simulink model "untitled"  (R2019a)
settings: Solver=VariableStepAuto  StartTime=0.0  StopTime=1  RelTol=1e-3
values from neighbouring files (symbols this model uses):
  Ts_Control = 5.0000e-05    (= 5e-05)    [Sec_Impedance.m]
  Ts_Power = 5.0000e-05    (= 5e-05)    [Sec_Impedance.m]
undefined symbols (not defined in the file or in its folder): D1, Delta, Ion, Lithium
libraries: powerlib x152, powerlib_meascontrol x65, simulink x14, electricdrivelib x12, simulink_extras x12
(part 3 of 5)

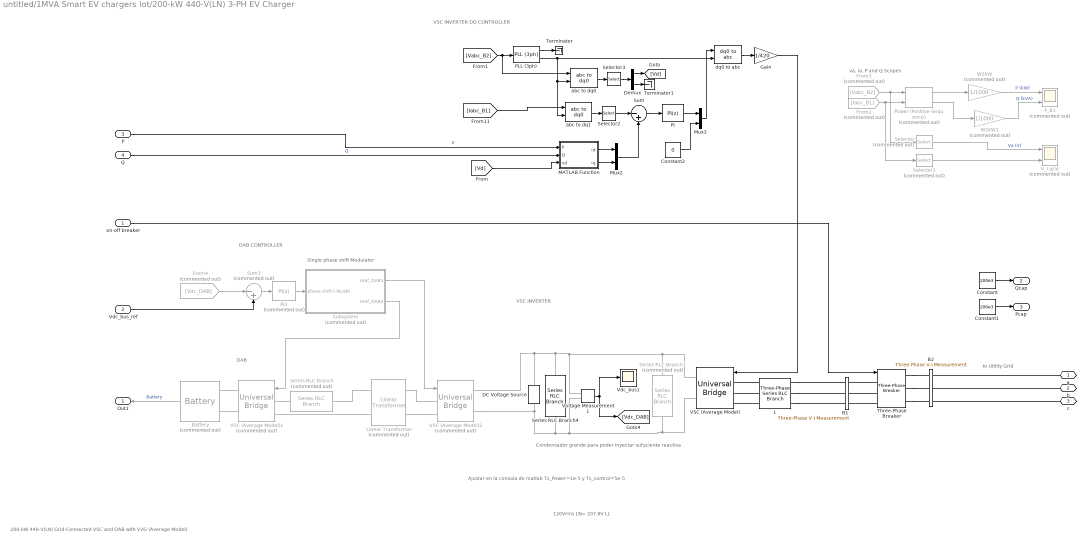
== system untitled/1MVA Smart EV chargers lot/200-kW 440-V(LN) 3-PH EV Charger ==
  note: DAB CONTROLLER
  note: va, ia, P and Q Scopes
  note: 200-kW 440-V(LN) Grid-Connected VSC and DAB with V2G (Average Model)
  note: 120Vrms LN= 207.8V LL
  note: Single phase shift Modulator
  note: Condensador grande para poder inyectar sufuciente reactiva
  note: Ajustar en la consola de matlab Ts_Power=1e-5 y Ts_control=5e-5
  note: to Utility Grid
  note: DAB
  note: VSC INVERTER
  note: VSC INVERTER DQ CONTROLLER
  on-off breaker : Inport
  Vdc_bus_ref : Inport  Port=2
  P : Inport  Port=3
  Q : Inport  Port=4
  B1 : powerlib/Measurements/Three-Phase V-I Measurement  VoltageMeasurement=no  SetLabelV=on  LabelV=Vabc_B1  Vpu=off  VpuLL=off  CurrentMeasurement=yes  SetLabelI=on  LabelI=Iabc_B1  Ipu=off  Pbase=100e6  Vbase=500e3  OutputType=Magnitude  PhasorSimulation=off  PSBequivalent=0
      settings: SourceProductName=Simscape Electrical
  B2 : powerlib/Measurements/Three-Phase V-I Measurement  VoltageMeasurement=phase-to-ground  SetLabelV=on  LabelV=Vabc_B2  Vpu=off  VpuLL=off  CurrentMeasurement=no  SetLabelI=off  LabelI=Iabc_B1  Ipu=off  Pbase=100e6  Vbase=500e3  OutputType=Magnitude  PhasorSimulation=off  PSBequivalent=0
      settings: SourceProductName=Simscape Electrical
  Battery : electricdrivelib/Extra Sources/Battery  Commented=on  BatType=Lithium-Ion  ShowTempParam=off  ThermalPreset=no  ShowAgeParam=off  NomV=380  NomQ=5.4*70  SOC=70  Batt_Tr=20  PresetModel=on  MaxQ=378  MinV=285  FullV=442.3151  Dis_rate=164.3478  R=0.010053  Normal_OP=341.8435  expZone="[410.5466       18.5713]"  current=[6.5 13 32.5]  Units=Time  Tci=20  NomT=20  T2=-30  MaxQ2=4.8  FullV2=7.1  Normal_OP2=5.655  expZone2="[6.58           1]"  Rca=0.6  ti=2000  Dp=0  Neq0=0  Tsim=1e6  Ta1=25  Qeol=5.4*0.9  Reol=0.013333*1.2  Char_age=[2.3478, 3]  Dis_age=[2.3478, 10]  N1=1500  N2=10500  N3=1000  N4=1400  Ta2=45  N5=950
      settings: SourceProductName=Simscape Electrical
  Constant : Constant  Value=200e3
  Constant1 : Constant  Value=200e3
  Constant2 : Constant  Value=0
  DC Voltage Source : powerlib/Electrical Sources/DC Voltage Source  Amplitude=800  Measurements=None
      settings: SourceProductName=Simscape Electrical
  Demux : Demux  Outputs=2
  From2 : From  Commented=on  GotoTag=Iabc_B1  TagVisibility=global
      settings: CloseFcn=tagdialog Close
  From3 : From  Commented=on  GotoTag=Vabc_B2  TagVisibility=global
      settings: CloseFcn=tagdialog Close
  From4 : From  Commented=on  GotoTag=Vdc_DAB
  Gain : Gain  Gain=1/420
  L : powerlib/Elements/Three-Phase Series RLC Branch  LConnTagsString=A|B|C  RConnTagsString=A|B|C  BranchType=RL  Resistance=500e-6*377/50/2  Inductance=1200e-6/2  Capacitance=inf  Measurements=None
      settings: SourceProductName=Simscape Electrical
  Linear Transformer : powerlib/Elements/Linear Transformer  Commented=on  UNITS=SI  NominalPower=[ 250e3 10000 ]  winding1=[400 0.0032 0.4883e-06]  winding2=[800 0.0032 0.4883e-06]  ThreeWindings=off  winding3=[3.15e+05 19845 2105.6]  RmLm=[800 2.1221]  Measurements=None  DataType=on
      settings: SourceProductName=Simscape Electrical
  MATLAB Function : MATLAB Function  TreatAsAtomicUnit=on
  Mux2 : Mux  Inputs=2
  Mux3 : Mux  Inputs=2
  PI : simulink/Continuous/PID Controller  Controller=PI  Form=Parallel  TimeDomain=Discrete-time  SampleTime=Ts_Control  IntegratorMethod=Forward Euler  FilterMethod=Forward Euler  ControllerParametersSource=internal  P=20  I=360  D=0  UseFilter=on  N=100  TunerSelectOption=Transfer Function Based (PID Tuner App)  InitialConditionSource=internal  InitialConditionForIntegrator=0  InitialConditionForFilter=0  DifferentiatorICPrevScaledInput=0  ExternalReset=none  TrackingMode=off  Kt=1  LimitOutput=on  UpperSaturationLimit=800  LowerSaturationLimit=-800  LinearizeAsGain=off  AntiWindupMode=none  Kb=1  POutMin=[]  POutMax=[]  IOutMin=[]  IOutMax=[]  DOutMin=[]  DOutMax=[]  NOutMin=[]  NOutMax=[]  SumOutMin=[]  SumOutMax=[]  SaturationOutMin=[]  SaturationOutMax=[]  PParamMin=[]  PParamMax=[]  IParamMin=[]  IParamMax=[]  DParamMin=[]  DParamMax=[]  NParamMin=[]  NParamMax=[]  KbParamMin=[]  KbParamMax=[]  KtParamMin=[]  KtParamMax=[]  KbOutMin=[]  KbOutMax=[]  KtOutMin=[]  KtOutMax=[]  IntegratorOutMin=[]  IntegratorOutMax=[]  FilterOutMin=[]  FilterOutMax=[]  SumI1OutMin=[]  SumI1OutMax=[]  SumI2OutMin=[]  SumI2OutMax=[]  SumI3OutMin=[]  SumI3OutMax=[]  SumI4OutMin=[]  SumI4OutMax=[]  SumDOutMin=[]  SumDOutMax=[]  DifferentiatorOutMin=[]  DifferentiatorOutMax=[]  FilterDiffOutCoefMin=[]  FilterDiffOutCoefMax=[]  ReciprocalOutMin=[]  ReciprocalOutMax=[]  SumDenOutMin=[]  SumDenOutMax=[]  SumNumOutMin=[]  SumNumOutMax=[]  DivideOutMin=[]  DivideOutMax=[]  IntegratorContinuousStateAttributes=''  IntegratorStateMustResolveToSignalObject=off  IntegratorRTWStateStorageClass=Auto  FilterContinuousStateAttributes=''  FilterStateMustResolveToSignalObject=off  FilterRTWStateStorageClass=Auto  ParallelPVariant=InternalParameters  IdealPVariant=Disabled  IVariant=InternalParameters  DVariant=Disabled  IntegratorVariant=Discrete  SatVariant=Enabled  AWVariant=Passthrough  PCopyVariant=Disabled  TRVariant=Disabled  FdbkBlocksVariant=Forward  IdealPFdbkVariant=Disabled  SatFdbkVariant=Disabled  DerivativeFilterVariant=Disabled  NVariant=Disabled  NCopyVariant=Disabled_SignalSpec  FilterICVariant=Disabled  IntegratorICVariant=InternalICs  ExternalResetVariant=Disabled  TRSumVariant=Passthrough  SumFdbkVariant=Disabled  SumVariant=Sum_PI
  PI3 : simulink/Continuous/PID Controller  Commented=on  Controller=PI  Form=Parallel  TimeDomain=Discrete-time  SampleTime=Ts_Control  IntegratorMethod=Forward Euler  FilterMethod=Forward Euler  ControllerParametersSource=internal  P=4  I=50  D=0  UseFilter=on  N=100  TunerSelectOption=Transfer Function Based (PID Tuner App)  InitialConditionSource=internal  InitialConditionForIntegrator=0  InitialConditionForFilter=0  DifferentiatorICPrevScaledInput=0  ExternalReset=none  TrackingMode=off  Kt=1  LimitOutput=on  UpperSaturationLimit=90  LowerSaturationLimit=-90  LinearizeAsGain=off  AntiWindupMode=none  Kb=1  POutMin=[]  POutMax=[]  IOutMin=[]  IOutMax=[]  DOutMin=[]  DOutMax=[]  NOutMin=[]  NOutMax=[]  SumOutMin=[]  SumOutMax=[]  SaturationOutMin=[]  SaturationOutMax=[]  PParamMin=[]  PParamMax=[]  IParamMin=[]  IParamMax=[]  DParamMin=[]  DParamMax=[]  NParamMin=[]  NParamMax=[]  KbParamMin=[]  KbParamMax=[]  KtParamMin=[]  KtParamMax=[]  KbOutMin=[]  KbOutMax=[]  KtOutMin=[]  KtOutMax=[]  IntegratorOutMin=[]  IntegratorOutMax=[]  FilterOutMin=[]  FilterOutMax=[]  SumI1OutMin=[]  SumI1OutMax=[]  SumI2OutMin=[]  SumI2OutMax=[]  SumI3OutMin=[]  SumI3OutMax=[]  SumI4OutMin=[]  SumI4OutMax=[]  SumDOutMin=[]  SumDOutMax=[]  DifferentiatorOutMin=[]  DifferentiatorOutMax=[]  FilterDiffOutCoefMin=[]  FilterDiffOutCoefMax=[]  ReciprocalOutMin=[]  ReciprocalOutMax=[]  SumDenOutMin=[]  SumDenOutMax=[]  SumNumOutMin=[]  SumNumOutMax=[]  DivideOutMin=[]  DivideOutMax=[]  IntegratorContinuousStateAttributes=''  IntegratorStateMustResolveToSignalObject=off  IntegratorRTWStateStorageClass=Auto  FilterContinuousStateAttributes=''  FilterStateMustResolveToSignalObject=off  FilterRTWStateStorageClass=Auto  ParallelPVariant=InternalParameters  IdealPVariant=Disabled  IVariant=InternalParameters  DVariant=Disabled  IntegratorVariant=Discrete  SatVariant=Enabled  AWVariant=Passthrough  PCopyVariant=Disabled  TRVariant=Disabled  FdbkBlocksVariant=Forward  IdealPFdbkVariant=Disabled  SatFdbkVariant=Disabled  DerivativeFilterVariant=Disabled  NVariant=Disabled  NCopyVariant=Disabled_SignalSpec  FilterICVariant=Disabled  IntegratorICVariant=InternalICs  ExternalResetVariant=Disabled  TRSumVariant=Passthrough  SumFdbkVariant=Disabled  SumVariant=Sum_PI
  PLL (3ph) : powerlib_meascontrol/PLL/PLL (3ph)  Fmin=58  Par_Init="[-0.57  60]"  ParK=[180, 3200, 1]  TcD=1e-4  MaxRateChangeFreq=12  FilterCutOffFreq=25  Ts=Ts_Power  AGC=on
      settings: SourceProductName=Simscape Electrical
  P_B1 : Scope  Commented=on  NumInputPorts=2
  Power (Positive-Sequence) : powerlib_meascontrol/Measurements/Power (Positive-Sequence)  Commented=on  Freq=60  Vinit=[0, 0]  Iinit=[0, 0]  Ts=Ts_Control
      settings: SourceProductName=Simscape Electrical  SourceProductBaseCode=PS
  Selector : Selector  Commented=on  InputPortWidth=3  IndexOptions=Index vector (dialog)  Indices=[1]  OutputSizes=1
  Selector1 : Selector  Commented=on  InputPortWidth=3  IndexOptions=Index vector (dialog)  Indices=[1]  OutputSizes=1
  Selector2 : Selector  InputPortWidth=3  IndexOptions=Index vector (dialog)  Indices=[1 2]  OutputSizes=1
  Selector3 : Selector  InputPortWidth=3  IndexOptions=Index vector (dialog)  Indices=[1 2]  OutputSizes=1
  Series RLC Branch : powerlib/Elements/Series RLC Branch  Commented=on  LConnTagsString=__new0  RConnTagsString=__new0  BranchType=L  Resistance=1  Inductance=1.5e-6  SetiL0=off  InitialCurrent=0  Capacitance=1e-6  Setx0=off  InitialVoltage=0  Measurements=None
      settings: SourceProductName=Simscape Electrical
  Series RLC Branch1 : powerlib/Elements/Series RLC Branch  Commented=on  LConnTagsString=__new0  RConnTagsString=__new0  BranchType=R  Resistance=3.2  Inductance=1e-3  SetiL0=off  InitialCurrent=0  Capacitance=1200e-6  Setx0=off  InitialVoltage=400  Measurements=None
      settings: SourceProductName=Simscape Electrical
  Series RLC Branch4 : powerlib/Elements/Series RLC Branch  LConnTagsString=__new0  RConnTagsString=__new0  BranchType=RC  Resistance=1e-7  Inductance=1e-3  SetiL0=off  InitialCurrent=0  Capacitance=3600e-6  Setx0=off  InitialVoltage=400  Measurements=None
      settings: SourceProductName=Simscape Electrical
  Subsystem : Subsystem  Commented=on
  Sum : Sum  Inputs=|-+
  Sum3 : Sum  Commented=on  Inputs=|-+
  Terminator : Terminator
  Terminator1 : Terminator
  Three-Phase Breaker : powerlib/Elements/Three-Phase Breaker  InitialState=open  SwitchA=on  SwitchB=on  SwitchC=on  SwitchTimes="[1/6  5/6]"  External=on  BreakerResistance=0.01e-3  SnubberResistance=30  SnubberCapacitance=20e-6  Measurements=None
      settings: SourceProductName=Simscape Electrical
  VSC (Average Model) : powerlib/Power Electronics/Universal Bridge  Arms=3  SnubberResistance=1e5  SnubberCapacitance=inf  Device=Average-model based VSC  Ron=1e-3  Lon=0  ForwardVoltages="[  0  0  ]"  ForwardVoltage=0  GTOparameters=[ 10e-6 , 20e-6 ]  IGBTparameters=[ 1e-6 , 2e-6 ]  Measurements=None  Measurements_2=None  converterType=Rectifier
      settings: SourceProductName=Simscape Electrical
  VSC (Average Model)1 : powerlib/Power Electronics/Universal Bridge  Commented=on  Arms=2  SnubberResistance=1e5  SnubberCapacitance=inf  Device=Average-model based VSC  Ron=1e-3  Lon=0  ForwardVoltages="[  0  0  ]"  ForwardVoltage=0  GTOparameters=[ 10e-6 , 20e-6 ]  IGBTparameters=[ 1e-6 , 2e-6 ]  Measurements=None  Measurements_2=None  converterType=Rectifier
      settings: SourceProductName=Simscape Electrical
  VSC (Average Model)2 : powerlib/Power Electronics/Universal Bridge  Commented=on  Arms=2  SnubberResistance=1e5  SnubberCapacitance=inf  Device=Average-model based VSC  Ron=1e-3  Lon=0  ForwardVoltages="[  0  0  ]"  ForwardVoltage=0  GTOparameters=[ 10e-6 , 20e-6 ]  IGBTparameters=[ 1e-6 , 2e-6 ]  Measurements=None  Measurements_2=None  converterType=Rectifier
      settings: SourceProductName=Simscape Electrical
  V_I grid : Scope  Commented=on  NumInputPorts=2
  Vdc_bus1 : Scope
  Voltage Measurement1 : powerlib/Measurements/Voltage Measurement  PhasorSimulation=off  OutputType=Complex  PSBequivalent=0
      settings: SourceProductName=Simscape Electrical
  W2kW : Gain  Commented=on  Gain=1/1000
  W2kW1 : Gain  Commented=on  Gain=1/1000
  abc to dq0 : powerlib_meascontrol/Transformations/abc to dq0  Alignment=90 degrees behind phase A axis
      settings: SourceProductName=Simscape Electrical
  abc to dq1 : powerlib_meascontrol/Transformations/abc to dq0  Alignment=90 degrees behind phase A axis
      settings: SourceProductName=Simscape Electrical
  dq0 to abc : powerlib_meascontrol/Transformations/dq0 to abc  Alignment=90 degrees behind phase A axis
      settings: SourceProductName=Simscape Electrical
  a : PMIOPort  Side=Right
  b : PMIOPort  Port=2  Side=Right
  c : PMIOPort  Port=3  Side=Right
  Out1 : Outport
  Qcap : Outport  Port=2
  Pcap : Outport  Port=3
  wires:
  PLL (3ph)/2 -> abc to dq1/2, abc to dq0/2, dq0 to abc/2
  Subsystem/1(Uref_DAB1) -> VSC (Average Model)2/1
  PI/1 -> Mux3/1
  Selector/1 -> V_I grid/1  "Va (V)"
  dq0 to abc/1 -> Gain/1
  Vdc_bus_ref/1 -> Sum3/2
  PLL (3ph)/1 -> Terminator/1
  From2/1 -> Selector1/1, Power (Positive-Sequence)/2
  abc to dq1/1 -> Selector2/1
  Mux3/1 -> dq0 to abc/1
  Gain/1 -> VSC (Average Model)/1
  W2kW1/1 -> P_B1/2  "Q (kVA)"
  Selector2/1 -> Sum/1
  Sum/1 -> PI/1
  [Vabc_B2] -> abc to dq0/1, PLL (3ph)/1
  Subsystem/2(Uref_DAB2) -> VSC (Average Model)1/1
  Sum3/1 -> PI3/1
  W2kW/1 -> P_B1/1  "P (kW)"
  Constant2/1 -> Mux3/2
  PI3/1 -> Subsystem/1(phase shift (-90,90))
  Selector3/1 -> Demux/1
  From3/1 -> Selector/1, Power (Positive-Sequence)/1
  Selector1/1 -> V_I grid/2
  From4/1 -> Sum3/1
  abc to dq0/1 -> Selector3/1
  Power (Positive-Sequence)/1 -> W2kW/1
  Voltage Measurement1/1 -> Vdc_bus1/1, [Vdc_DAB]
  Mux2/1 -> Sum/2
  [Iabc_B1] -> abc to dq1/1
  Power (Positive-Sequence)/2 -> W2kW1/1
  Battery/1 -> Out1/1  "Battery"
  on-off breaker/1 -> Three-Phase Breaker/1
  Demux/2 -> Terminator1/1
  Demux/1 -> [Vd]
  MATLAB Function/1(id) -> Mux2/1
  MATLAB Function/2(iq) -> Mux2/2
  [Vd] -> MATLAB Function/3(vd)
  P/1 -> MATLAB Function/1(P)  "P"
  Q/1 -> MATLAB Function/2(Q)  "Q"
  Constant1/1 -> Pcap/1
  Constant/1 -> Qcap/1
  connections:
  Battery/LConn1 -- VSC (Average Model)1/RConn1
  Three-Phase Breaker/LConn1 -- B1/RConn1
  Three-Phase Breaker/RConn2 -- B2/LConn2
  VSC (Average Model)2/RConn2 -- DC Voltage Source/LConn1 -- Series RLC Branch4/RConn1 -- Voltage Measurement1/LConn2 -- VSC (Average Model)/RConn2 -- Series RLC Branch1/RConn1
  L/RConn3 -- B1/LConn3
  L/LConn1 -- VSC (Average Model)/LConn1
  L/RConn1 -- B1/LConn1
  L/LConn2 -- VSC (Average Model)/LConn2
  VSC (Average Model)2/RConn1 -- Series RLC Branch1/LConn1 -- VSC (Average Model)/RConn1 -- Voltage Measurement1/LConn1 -- Series RLC Branch4/LConn1 -- DC Voltage Source/RConn1
  Series RLC Branch/RConn1 -- Linear Transformer/LConn1
  Linear Transformer/LConn2 -- VSC (Average Model)1/LConn2
  Three-Phase Breaker/LConn2 -- B1/RConn2
  VSC (Average Model)1/RConn2 -- Battery/LConn2
  Three-Phase Breaker/RConn3 -- B2/LConn3
  Three-Phase Breaker/RConn1 -- B2/LConn1
  Linear Transformer/RConn1 -- VSC (Average Model)2/LConn1
  Linear Transformer/RConn2 -- VSC (Average Model)2/LConn2
  c/RConn1 -- B2/RConn3
  Series RLC Branch/LConn1 -- VSC (Average Model)1/LConn1
  L/RConn2 -- B1/LConn2
  L/LConn3 -- VSC (Average Model)/LConn3
  Three-Phase Breaker/LConn3 -- B1/RConn3
  b/RConn1 -- B2/RConn2
  a/RConn1 -- B2/RConn1

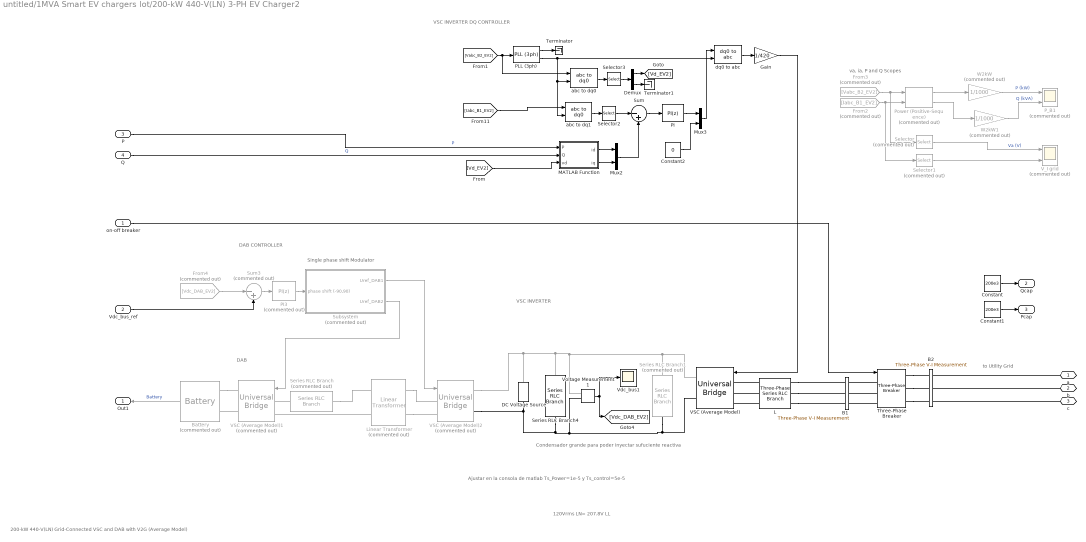
== system untitled/1MVA Smart EV chargers lot/200-kW 440-V(LN) 3-PH EV Charger2 ==
  note: DAB CONTROLLER
  note: va, ia, P and Q Scopes
  note: 200-kW 440-V(LN) Grid-Connected VSC and DAB with V2G (Average Model)
  note: 120Vrms LN= 207.8V LL
  note: Single phase shift Modulator
  note: Condensador grande para poder inyectar sufuciente reactiva
  note: Ajustar en la consola de matlab Ts_Power=1e-5 y Ts_control=5e-5
  note: to Utility Grid
  note: DAB
  note: VSC INVERTER
  note: VSC INVERTER DQ CONTROLLER
  on-off breaker : Inport
  Vdc_bus_ref : Inport  Port=2
  P : Inport  Port=3
  Q : Inport  Port=4
  B1 : powerlib/Measurements/Three-Phase V-I Measurement  VoltageMeasurement=no  SetLabelV=on  LabelV=Vabc_B1  Vpu=off  VpuLL=off  CurrentMeasurement=yes  SetLabelI=on  LabelI=Iabc_B1_EV2  Ipu=off  Pbase=100e6  Vbase=500e3  OutputType=Magnitude  PhasorSimulation=off  PSBequivalent=0
      settings: SourceProductName=Simscape Electrical
  B2 : powerlib/Measurements/Three-Phase V-I Measurement  VoltageMeasurement=phase-to-ground  SetLabelV=on  LabelV=Vabc_B2_EV2  Vpu=off  VpuLL=off  CurrentMeasurement=no  SetLabelI=off  LabelI=Iabc_B1  Ipu=off  Pbase=100e6  Vbase=500e3  OutputType=Magnitude  PhasorSimulation=off  PSBequivalent=0
      settings: SourceProductName=Simscape Electrical
  Battery : electricdrivelib/Extra Sources/Battery  Commented=on  BatType=Lithium-Ion  ShowTempParam=off  ThermalPreset=no  ShowAgeParam=off  NomV=380  NomQ=5.4*70  SOC=70  Batt_Tr=20  PresetModel=on  MaxQ=378  MinV=285  FullV=442.3151  Dis_rate=164.3478  R=0.010053  Normal_OP=341.8435  expZone="[410.5466       18.5713]"  current=[6.5 13 32.5]  Units=Time  Tci=20  NomT=20  T2=-30  MaxQ2=4.8  FullV2=7.1  Normal_OP2=5.655  expZone2="[6.58           1]"  Rca=0.6  ti=2000  Dp=0  Neq0=0  Tsim=1e6  Ta1=25  Qeol=5.4*0.9  Reol=0.013333*1.2  Char_age=[2.3478, 3]  Dis_age=[2.3478, 10]  N1=1500  N2=10500  N3=1000  N4=1400  Ta2=45  N5=950
      settings: SourceProductName=Simscape Electrical
  Constant : Constant  Value=200e3
  Constant1 : Constant  Value=200e3
  Constant2 : Constant  Value=0
  DC Voltage Source : powerlib/Electrical Sources/DC Voltage Source  Amplitude=800  Measurements=None
      settings: SourceProductName=Simscape Electrical
  Demux : Demux  Outputs=2
  From2 : From  Commented=on  GotoTag=Iabc_B1_EV2  TagVisibility=global
      settings: CloseFcn=tagdialog Close
  From3 : From  Commented=on  GotoTag=Vabc_B2_EV2  TagVisibility=global
      settings: CloseFcn=tagdialog Close
  From4 : From  Commented=on  GotoTag=Vdc_DAB_EV2
  Gain : Gain  Gain=1/420
  L : powerlib/Elements/Three-Phase Series RLC Branch  LConnTagsString=A|B|C  RConnTagsString=A|B|C  BranchType=RL  Resistance=500e-6*377/50/2  Inductance=1200e-6/2  Capacitance=inf  Measurements=None
      settings: SourceProductName=Simscape Electrical
  Linear Transformer : powerlib/Elements/Linear Transformer  Commented=on  UNITS=SI  NominalPower=[ 250e3 10000 ]  winding1=[400 0.0032 0.4883e-06]  winding2=[800 0.0032 0.4883e-06]  ThreeWindings=off  winding3=[3.15e+05 19845 2105.6]  RmLm=[800 2.1221]  Measurements=None  DataType=on
      settings: SourceProductName=Simscape Electrical
  MATLAB Function : MATLAB Function  TreatAsAtomicUnit=on
  Mux2 : Mux  Inputs=2
  Mux3 : Mux  Inputs=2
  PI : simulink/Continuous/PID Controller  Controller=PI  Form=Parallel  TimeDomain=Discrete-time  SampleTime=Ts_Control  IntegratorMethod=Forward Euler  FilterMethod=Forward Euler  ControllerParametersSource=internal  P=20  I=360  D=0  UseFilter=on  N=100  TunerSelectOption=Transfer Function Based (PID Tuner App)  InitialConditionSource=internal  InitialConditionForIntegrator=0  InitialConditionForFilter=0  DifferentiatorICPrevScaledInput=0  ExternalReset=none  TrackingMode=off  Kt=1  LimitOutput=on  UpperSaturationLimit=800  LowerSaturationLimit=-800  LinearizeAsGain=off  AntiWindupMode=none  Kb=1  POutMin=[]  POutMax=[]  IOutMin=[]  IOutMax=[]  DOutMin=[]  DOutMax=[]  NOutMin=[]  NOutMax=[]  SumOutMin=[]  SumOutMax=[]  SaturationOutMin=[]  SaturationOutMax=[]  PParamMin=[]  PParamMax=[]  IParamMin=[]  IParamMax=[]  DParamMin=[]  DParamMax=[]  NParamMin=[]  NParamMax=[]  KbParamMin=[]  KbParamMax=[]  KtParamMin=[]  KtParamMax=[]  KbOutMin=[]  KbOutMax=[]  KtOutMin=[]  KtOutMax=[]  IntegratorOutMin=[]  IntegratorOutMax=[]  FilterOutMin=[]  FilterOutMax=[]  SumI1OutMin=[]  SumI1OutMax=[]  SumI2OutMin=[]  SumI2OutMax=[]  SumI3OutMin=[]  SumI3OutMax=[]  SumI4OutMin=[]  SumI4OutMax=[]  SumDOutMin=[]  SumDOutMax=[]  DifferentiatorOutMin=[]  DifferentiatorOutMax=[]  FilterDiffOutCoefMin=[]  FilterDiffOutCoefMax=[]  ReciprocalOutMin=[]  ReciprocalOutMax=[]  SumDenOutMin=[]  SumDenOutMax=[]  SumNumOutMin=[]  SumNumOutMax=[]  DivideOutMin=[]  DivideOutMax=[]  IntegratorContinuousStateAttributes=''  IntegratorStateMustResolveToSignalObject=off  IntegratorRTWStateStorageClass=Auto  FilterContinuousStateAttributes=''  FilterStateMustResolveToSignalObject=off  FilterRTWStateStorageClass=Auto  ParallelPVariant=InternalParameters  IdealPVariant=Disabled  IVariant=InternalParameters  DVariant=Disabled  IntegratorVariant=Discrete  SatVariant=Enabled  AWVariant=Passthrough  PCopyVariant=Disabled  TRVariant=Disabled  FdbkBlocksVariant=Forward  IdealPFdbkVariant=Disabled  SatFdbkVariant=Disabled  DerivativeFilterVariant=Disabled  NVariant=Disabled  NCopyVariant=Disabled_SignalSpec  FilterICVariant=Disabled  IntegratorICVariant=InternalICs  ExternalResetVariant=Disabled  TRSumVariant=Passthrough  SumFdbkVariant=Disabled  SumVariant=Sum_PI
  PI3 : simulink/Continuous/PID Controller  Commented=on  Controller=PI  Form=Parallel  TimeDomain=Discrete-time  SampleTime=Ts_Control  IntegratorMethod=Forward Euler  FilterMethod=Forward Euler  ControllerParametersSource=internal  P=4  I=50  D=0  UseFilter=on  N=100  TunerSelectOption=Transfer Function Based (PID Tuner App)  InitialConditionSource=internal  InitialConditionForIntegrator=0  InitialConditionForFilter=0  DifferentiatorICPrevScaledInput=0  ExternalReset=none  TrackingMode=off  Kt=1  LimitOutput=on  UpperSaturationLimit=90  LowerSaturationLimit=-90  LinearizeAsGain=off  AntiWindupMode=none  Kb=1  POutMin=[]  POutMax=[]  IOutMin=[]  IOutMax=[]  DOutMin=[]  DOutMax=[]  NOutMin=[]  NOutMax=[]  SumOutMin=[]  SumOutMax=[]  SaturationOutMin=[]  SaturationOutMax=[]  PParamMin=[]  PParamMax=[]  IParamMin=[]  IParamMax=[]  DParamMin=[]  DParamMax=[]  NParamMin=[]  NParamMax=[]  KbParamMin=[]  KbParamMax=[]  KtParamMin=[]  KtParamMax=[]  KbOutMin=[]  KbOutMax=[]  KtOutMin=[]  KtOutMax=[]  IntegratorOutMin=[]  IntegratorOutMax=[]  FilterOutMin=[]  FilterOutMax=[]  SumI1OutMin=[]  SumI1OutMax=[]  SumI2OutMin=[]  SumI2OutMax=[]  SumI3OutMin=[]  SumI3OutMax=[]  SumI4OutMin=[]  SumI4OutMax=[]  SumDOutMin=[]  SumDOutMax=[]  DifferentiatorOutMin=[]  DifferentiatorOutMax=[]  FilterDiffOutCoefMin=[]  FilterDiffOutCoefMax=[]  ReciprocalOutMin=[]  ReciprocalOutMax=[]  SumDenOutMin=[]  SumDenOutMax=[]  SumNumOutMin=[]  SumNumOutMax=[]  DivideOutMin=[]  DivideOutMax=[]  IntegratorContinuousStateAttributes=''  IntegratorStateMustResolveToSignalObject=off  IntegratorRTWStateStorageClass=Auto  FilterContinuousStateAttributes=''  FilterStateMustResolveToSignalObject=off  FilterRTWStateStorageClass=Auto  ParallelPVariant=InternalParameters  IdealPVariant=Disabled  IVariant=InternalParameters  DVariant=Disabled  IntegratorVariant=Discrete  SatVariant=Enabled  AWVariant=Passthrough  PCopyVariant=Disabled  TRVariant=Disabled  FdbkBlocksVariant=Forward  IdealPFdbkVariant=Disabled  SatFdbkVariant=Disabled  DerivativeFilterVariant=Disabled  NVariant=Disabled  NCopyVariant=Disabled_SignalSpec  FilterICVariant=Disabled  IntegratorICVariant=InternalICs  ExternalResetVariant=Disabled  TRSumVariant=Passthrough  SumFdbkVariant=Disabled  SumVariant=Sum_PI
  PLL (3ph) : powerlib_meascontrol/PLL/PLL (3ph)  Fmin=55  Par_Init="[-0.57  60]"  ParK=[180, 3200, 1]  TcD=1e-4  MaxRateChangeFreq=12  FilterCutOffFreq=25  Ts=Ts_Power  AGC=on
      settings: SourceProductName=Simscape Electrical
  P_B1 : Scope  Commented=on  NumInputPorts=2
  Power (Positive-Sequence) : powerlib_meascontrol/Measurements/Power (Positive-Sequence)  Commented=on  Freq=60  Vinit=[0, 0]  Iinit=[0, 0]  Ts=Ts_Control
      settings: SourceProductName=Simscape Electrical  SourceProductBaseCode=PS
  Selector : Selector  Commented=on  InputPortWidth=3  IndexOptions=Index vector (dialog)  Indices=[1]  OutputSizes=1
  Selector1 : Selector  Commented=on  InputPortWidth=3  IndexOptions=Index vector (dialog)  Indices=[1]  OutputSizes=1
  Selector2 : Selector  InputPortWidth=3  IndexOptions=Index vector (dialog)  Indices=[1 2]  OutputSizes=1
  Selector3 : Selector  InputPortWidth=3  IndexOptions=Index vector (dialog)  Indices=[1 2]  OutputSizes=1
  Series RLC Branch : powerlib/Elements/Series RLC Branch  Commented=on  LConnTagsString=__new0  RConnTagsString=__new0  BranchType=L  Resistance=1  Inductance=1.5e-6  SetiL0=off  InitialCurrent=0  Capacitance=1e-6  Setx0=off  InitialVoltage=0  Measurements=None
      settings: SourceProductName=Simscape Electrical
  Series RLC Branch1 : powerlib/Elements/Series RLC Branch  Commented=on  LConnTagsString=__new0  RConnTagsString=__new0  BranchType=R  Resistance=3.2  Inductance=1e-3  SetiL0=off  InitialCurrent=0  Capacitance=1200e-6  Setx0=off  InitialVoltage=400  Measurements=None
      settings: SourceProductName=Simscape Electrical
  Series RLC Branch4 : powerlib/Elements/Series RLC Branch  LConnTagsString=__new0  RConnTagsString=__new0  BranchType=RC  Resistance=1e-7  Inductance=1e-3  SetiL0=off  InitialCurrent=0  Capacitance=3600e-6  Setx0=off  InitialVoltage=400  Measurements=None
      settings: SourceProductName=Simscape Electrical
  Subsystem : Subsystem  Commented=on
  Sum : Sum  Inputs=|-+
  Sum3 : Sum  Commented=on  Inputs=|-+
  Terminator : Terminator
  Terminator1 : Terminator
  Three-Phase Breaker : powerlib/Elements/Three-Phase Breaker  InitialState=open  SwitchA=on  SwitchB=on  SwitchC=on  SwitchTimes="[1/6  5/6]"  External=on  BreakerResistance=0.01e-3  SnubberResistance=30  SnubberCapacitance=20e-6  Measurements=None
      settings: SourceProductName=Simscape Electrical
  VSC (Average Model) : powerlib/Power Electronics/Universal Bridge  Arms=3  SnubberResistance=1e5  SnubberCapacitance=inf  Device=Average-model based VSC  Ron=1e-3  Lon=0  ForwardVoltages="[  0  0  ]"  ForwardVoltage=0  GTOparameters=[ 10e-6 , 20e-6 ]  IGBTparameters=[ 1e-6 , 2e-6 ]  Measurements=None  Measurements_2=None  converterType=Rectifier
      settings: SourceProductName=Simscape Electrical
  VSC (Average Model)1 : powerlib/Power Electronics/Universal Bridge  Commented=on  Arms=2  SnubberResistance=1e5  SnubberCapacitance=inf  Device=Average-model based VSC  Ron=1e-3  Lon=0  ForwardVoltages="[  0  0  ]"  ForwardVoltage=0  GTOparameters=[ 10e-6 , 20e-6 ]  IGBTparameters=[ 1e-6 , 2e-6 ]  Measurements=None  Measurements_2=None  converterType=Rectifier
      settings: SourceProductName=Simscape Electrical
  VSC (Average Model)2 : powerlib/Power Electronics/Universal Bridge  Commented=on  Arms=2  SnubberResistance=1e5  SnubberCapacitance=inf  Device=Average-model based VSC  Ron=1e-3  Lon=0  ForwardVoltages="[  0  0  ]"  ForwardVoltage=0  GTOparameters=[ 10e-6 , 20e-6 ]  IGBTparameters=[ 1e-6 , 2e-6 ]  Measurements=None  Measurements_2=None  converterType=Rectifier
      settings: SourceProductName=Simscape Electrical
  V_I grid : Scope  Commented=on  NumInputPorts=2
  Vdc_bus1 : Scope
  Voltage Measurement1 : powerlib/Measurements/Voltage Measurement  PhasorSimulation=off  OutputType=Complex  PSBequivalent=0
      settings: SourceProductName=Simscape Electrical
  W2kW : Gain  Commented=on  Gain=1/1000
  W2kW1 : Gain  Commented=on  Gain=1/1000
  abc to dq0 : powerlib_meascontrol/Transformations/abc to dq0  Alignment=90 degrees behind phase A axis
      settings: SourceProductName=Simscape Electrical
  abc to dq1 : powerlib_meascontrol/Transformations/abc to dq0  Alignment=90 degrees behind phase A axis
      settings: SourceProductName=Simscape Electrical
  dq0 to abc : powerlib_meascontrol/Transformations/dq0 to abc  Alignment=90 degrees behind phase A axis
      settings: SourceProductName=Simscape Electrical
  a : PMIOPort  Side=Right
  b : PMIOPort  Port=2  Side=Right
  c : PMIOPort  Port=3  Side=Right
  Out1 : Outport
  Qcap : Outport  Port=2
  Pcap : Outport  Port=3
  wires:
  PLL (3ph)/2 -> abc to dq1/2, abc to dq0/2, dq0 to abc/2
  Subsystem/1(Uref_DAB1) -> VSC (Average Model)2/1
  PI/1 -> Mux3/1
  Selector/1 -> V_I grid/1  "Va (V)"
  dq0 to abc/1 -> Gain/1
  Vdc_bus_ref/1 -> Sum3/2
  PLL (3ph)/1 -> Terminator/1
  From2/1 -> Selector1/1, Power (Positive-Sequence)/2
  abc to dq1/1 -> Selector2/1
  Mux3/1 -> dq0 to abc/1
  Gain/1 -> VSC (Average Model)/1
  W2kW1/1 -> P_B1/2  "Q (kVA)"
  Selector2/1 -> Sum/1
  Sum/1 -> PI/1
  [Vabc_B2_EV2] -> abc to dq0/1, PLL (3ph)/1
  Subsystem/2(Uref_DAB2) -> VSC (Average Model)1/1
  Sum3/1 -> PI3/1
  W2kW/1 -> P_B1/1  "P (kW)"
  Constant2/1 -> Mux3/2
  PI3/1 -> Subsystem/1(phase shift (-90,90))
  Selector3/1 -> Demux/1
  From3/1 -> Selector/1, Power (Positive-Sequence)/1
  Selector1/1 -> V_I grid/2
  From4/1 -> Sum3/1
  abc to dq0/1 -> Selector3/1
  Power (Positive-Sequence)/1 -> W2kW/1
  Voltage Measurement1/1 -> Vdc_bus1/1, [Vdc_DAB_EV2]
  Mux2/1 -> Sum/2
  [Iabc_B1_EV2] -> abc to dq1/1
  Power (Positive-Sequence)/2 -> W2kW1/1
  Battery/1 -> Out1/1  "Battery"
  on-off breaker/1 -> Three-Phase Breaker/1
  Demux/2 -> Terminator1/1
  Demux/1 -> [Vd_EV2]
  MATLAB Function/1(id) -> Mux2/1
  MATLAB Function/2(iq) -> Mux2/2
  [Vd_EV2] -> MATLAB Function/3(vd)
  P/1 -> MATLAB Function/1(P)  "P"
  Q/1 -> MATLAB Function/2(Q)  "Q"
  Constant1/1 -> Pcap/1
  Constant/1 -> Qcap/1
  connections:
  Battery/LConn1 -- VSC (Average Model)1/RConn1
  Three-Phase Breaker/LConn1 -- B1/RConn1
  Three-Phase Breaker/RConn2 -- B2/LConn2
  VSC (Average Model)/RConn2 -- Series RLC Branch1/RConn1 -- VSC (Average Model)2/RConn2 -- DC Voltage Source/LConn1 -- Series RLC Branch4/RConn1 -- Voltage Measurement1/LConn2
  L/RConn3 -- B1/LConn3
  L/LConn1 -- VSC (Average Model)/LConn1
  L/RConn1 -- B1/LConn1
  L/LConn2 -- VSC (Average Model)/LConn2
  Series RLC Branch1/LConn1 -- VSC (Average Model)/RConn1 -- DC Voltage Source/RConn1 -- VSC (Average Model)2/RConn1 -- Series RLC Branch4/LConn1 -- Voltage Measurement1/LConn1
  Series RLC Branch/RConn1 -- Linear Transformer/LConn1
  Linear Transformer/LConn2 -- VSC (Average Model)1/LConn2
  Three-Phase Breaker/LConn2 -- B1/RConn2
  VSC (Average Model)1/RConn2 -- Battery/LConn2
  Three-Phase Breaker/RConn3 -- B2/LConn3
  Three-Phase Breaker/RConn1 -- B2/LConn1
  Linear Transformer/RConn1 -- VSC (Average Model)2/LConn1
  Linear Transformer/RConn2 -- VSC (Average Model)2/LConn2
  c/RConn1 -- B2/RConn3
  Series RLC Branch/LConn1 -- VSC (Average Model)1/LConn1
  L/RConn2 -- B1/LConn2
  L/LConn3 -- VSC (Average Model)/LConn3
  Three-Phase Breaker/LConn3 -- B1/RConn3
  b/RConn1 -- B2/RConn2
  a/RConn1 -- B2/RConn1

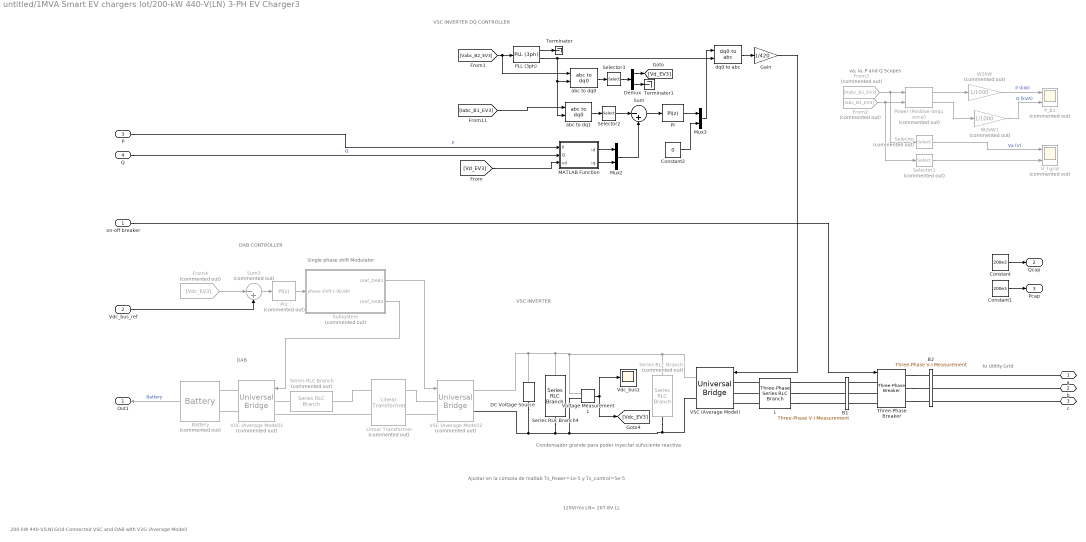
== system untitled/1MVA Smart EV chargers lot/200-kW 440-V(LN) 3-PH EV Charger3 ==
  note: DAB CONTROLLER
  note: va, ia, P and Q Scopes
  note: 200-kW 440-V(LN) Grid-Connected VSC and DAB with V2G (Average Model)
  note: 120Vrms LN= 207.8V LL
  note: Single phase shift Modulator
  note: Condensador grande para poder inyectar sufuciente reactiva
  note: Ajustar en la consola de matlab Ts_Power=1e-5 y Ts_control=5e-5
  note: to Utility Grid
  note: DAB
  note: VSC INVERTER
  note: VSC INVERTER DQ CONTROLLER
  on-off breaker : Inport
  Vdc_bus_ref : Inport  Port=2
  P : Inport  Port=3
  Q : Inport  Port=4
  B1 : powerlib/Measurements/Three-Phase V-I Measurement  VoltageMeasurement=no  SetLabelV=on  LabelV=Vabc_B1  Vpu=off  VpuLL=off  CurrentMeasurement=yes  SetLabelI=on  LabelI=Iabc_B1_EV3  Ipu=off  Pbase=100e6  Vbase=500e3  OutputType=Magnitude  PhasorSimulation=off  PSBequivalent=0
      settings: SourceProductName=Simscape Electrical
  B2 : powerlib/Measurements/Three-Phase V-I Measurement  VoltageMeasurement=phase-to-ground  SetLabelV=on  LabelV=Vabc_B2_EV3  Vpu=off  VpuLL=off  CurrentMeasurement=no  SetLabelI=off  LabelI=Iabc_B1  Ipu=off  Pbase=100e6  Vbase=500e3  OutputType=Magnitude  PhasorSimulation=off  PSBequivalent=0
      settings: SourceProductName=Simscape Electrical
  Battery : electricdrivelib/Extra Sources/Battery  Commented=on  BatType=Lithium-Ion  ShowTempParam=off  ThermalPreset=no  ShowAgeParam=off  NomV=380  NomQ=5.4*70  SOC=70  Batt_Tr=20  PresetModel=on  MaxQ=378  MinV=285  FullV=442.3151  Dis_rate=164.3478  R=0.010053  Normal_OP=341.8435  expZone="[410.5466       18.5713]"  current=[6.5 13 32.5]  Units=Time  Tci=20  NomT=20  T2=-30  MaxQ2=4.8  FullV2=7.1  Normal_OP2=5.655  expZone2="[6.58           1]"  Rca=0.6  ti=2000  Dp=0  Neq0=0  Tsim=1e6  Ta1=25  Qeol=5.4*0.9  Reol=0.013333*1.2  Char_age=[2.3478, 3]  Dis_age=[2.3478, 10]  N1=1500  N2=10500  N3=1000  N4=1400  Ta2=45  N5=950
      settings: SourceProductName=Simscape Electrical
  Constant : Constant  Value=200e3
  Constant1 : Constant  Value=200e3
  Constant2 : Constant  Value=0
  DC Voltage Source : powerlib/Electrical Sources/DC Voltage Source  Amplitude=800  Measurements=None
      settings: SourceProductName=Simscape Electrical
  Demux : Demux  Outputs=2
  From2 : From  Commented=on  GotoTag=Iabc_B1_EV3  TagVisibility=global
      settings: CloseFcn=tagdialog Close
  From3 : From  Commented=on  GotoTag=Vabc_B2_EV3  TagVisibility=global
      settings: CloseFcn=tagdialog Close
  From4 : From  Commented=on  GotoTag=Vdc_EV3
  Gain : Gain  Gain=1/420
  L : powerlib/Elements/Three-Phase Series RLC Branch  LConnTagsString=A|B|C  RConnTagsString=A|B|C  BranchType=RL  Resistance=500e-6*377/50/2  Inductance=1200e-6/2  Capacitance=inf  Measurements=None
      settings: SourceProductName=Simscape Electrical
  Linear Transformer : powerlib/Elements/Linear Transformer  Commented=on  UNITS=SI  NominalPower=[ 250e3 10000 ]  winding1=[400 0.0032 0.4883e-06]  winding2=[800 0.0032 0.4883e-06]  ThreeWindings=off  winding3=[3.15e+05 19845 2105.6]  RmLm=[800 2.1221]  Measurements=None  DataType=on
      settings: SourceProductName=Simscape Electrical
  MATLAB Function : MATLAB Function  TreatAsAtomicUnit=on
  Mux2 : Mux  Inputs=2
  Mux3 : Mux  Inputs=2
  PI : simulink/Continuous/PID Controller  Controller=PI  Form=Parallel  TimeDomain=Discrete-time  SampleTime=Ts_Control  IntegratorMethod=Forward Euler  FilterMethod=Forward Euler  ControllerParametersSource=internal  P=20  I=360  D=0  UseFilter=on  N=100  TunerSelectOption=Transfer Function Based (PID Tuner App)  InitialConditionSource=internal  InitialConditionForIntegrator=0  InitialConditionForFilter=0  DifferentiatorICPrevScaledInput=0  ExternalReset=none  TrackingMode=off  Kt=1  LimitOutput=on  UpperSaturationLimit=800  LowerSaturationLimit=-800  LinearizeAsGain=off  AntiWindupMode=none  Kb=1  POutMin=[]  POutMax=[]  IOutMin=[]  IOutMax=[]  DOutMin=[]  DOutMax=[]  NOutMin=[]  NOutMax=[]  SumOutMin=[]  SumOutMax=[]  SaturationOutMin=[]  SaturationOutMax=[]  PParamMin=[]  PParamMax=[]  IParamMin=[]  IParamMax=[]  DParamMin=[]  DParamMax=[]  NParamMin=[]  NParamMax=[]  KbParamMin=[]  KbParamMax=[]  KtParamMin=[]  KtParamMax=[]  KbOutMin=[]  KbOutMax=[]  KtOutMin=[]  KtOutMax=[]  IntegratorOutMin=[]  IntegratorOutMax=[]  FilterOutMin=[]  FilterOutMax=[]  SumI1OutMin=[]  SumI1OutMax=[]  SumI2OutMin=[]  SumI2OutMax=[]  SumI3OutMin=[]  SumI3OutMax=[]  SumI4OutMin=[]  SumI4OutMax=[]  SumDOutMin=[]  SumDOutMax=[]  DifferentiatorOutMin=[]  DifferentiatorOutMax=[]  FilterDiffOutCoefMin=[]  FilterDiffOutCoefMax=[]  ReciprocalOutMin=[]  ReciprocalOutMax=[]  SumDenOutMin=[]  SumDenOutMax=[]  SumNumOutMin=[]  SumNumOutMax=[]  DivideOutMin=[]  DivideOutMax=[]  IntegratorContinuousStateAttributes=''  IntegratorStateMustResolveToSignalObject=off  IntegratorRTWStateStorageClass=Auto  FilterContinuousStateAttributes=''  FilterStateMustResolveToSignalObject=off  FilterRTWStateStorageClass=Auto  ParallelPVariant=InternalParameters  IdealPVariant=Disabled  IVariant=InternalParameters  DVariant=Disabled  IntegratorVariant=Discrete  SatVariant=Enabled  AWVariant=Passthrough  PCopyVariant=Disabled  TRVariant=Disabled  FdbkBlocksVariant=Forward  IdealPFdbkVariant=Disabled  SatFdbkVariant=Disabled  DerivativeFilterVariant=Disabled  NVariant=Disabled  NCopyVariant=Disabled_SignalSpec  FilterICVariant=Disabled  IntegratorICVariant=InternalICs  ExternalResetVariant=Disabled  TRSumVariant=Passthrough  SumFdbkVariant=Disabled  SumVariant=Sum_PI
  PI3 : simulink/Continuous/PID Controller  Commented=on  Controller=PI  Form=Parallel  TimeDomain=Discrete-time  SampleTime=Ts_Control  IntegratorMethod=Forward Euler  FilterMethod=Forward Euler  ControllerParametersSource=internal  P=4  I=50  D=0  UseFilter=on  N=100  TunerSelectOption=Transfer Function Based (PID Tuner App)  InitialConditionSource=internal  InitialConditionForIntegrator=0  InitialConditionForFilter=0  DifferentiatorICPrevScaledInput=0  ExternalReset=none  TrackingMode=off  Kt=1  LimitOutput=on  UpperSaturationLimit=90  LowerSaturationLimit=-90  LinearizeAsGain=off  AntiWindupMode=none  Kb=1  POutMin=[]  POutMax=[]  IOutMin=[]  IOutMax=[]  DOutMin=[]  DOutMax=[]  NOutMin=[]  NOutMax=[]  SumOutMin=[]  SumOutMax=[]  SaturationOutMin=[]  SaturationOutMax=[]  PParamMin=[]  PParamMax=[]  IParamMin=[]  IParamMax=[]  DParamMin=[]  DParamMax=[]  NParamMin=[]  NParamMax=[]  KbParamMin=[]  KbParamMax=[]  KtParamMin=[]  KtParamMax=[]  KbOutMin=[]  KbOutMax=[]  KtOutMin=[]  KtOutMax=[]  IntegratorOutMin=[]  IntegratorOutMax=[]  FilterOutMin=[]  FilterOutMax=[]  SumI1OutMin=[]  SumI1OutMax=[]  SumI2OutMin=[]  SumI2OutMax=[]  SumI3OutMin=[]  SumI3OutMax=[]  SumI4OutMin=[]  SumI4OutMax=[]  SumDOutMin=[]  SumDOutMax=[]  DifferentiatorOutMin=[]  DifferentiatorOutMax=[]  FilterDiffOutCoefMin=[]  FilterDiffOutCoefMax=[]  ReciprocalOutMin=[]  ReciprocalOutMax=[]  SumDenOutMin=[]  SumDenOutMax=[]  SumNumOutMin=[]  SumNumOutMax=[]  DivideOutMin=[]  DivideOutMax=[]  IntegratorContinuousStateAttributes=''  IntegratorStateMustResolveToSignalObject=off  IntegratorRTWStateStorageClass=Auto  FilterContinuousStateAttributes=''  FilterStateMustResolveToSignalObject=off  FilterRTWStateStorageClass=Auto  ParallelPVariant=InternalParameters  IdealPVariant=Disabled  IVariant=InternalParameters  DVariant=Disabled  IntegratorVariant=Discrete  SatVariant=Enabled  AWVariant=Passthrough  PCopyVariant=Disabled  TRVariant=Disabled  FdbkBlocksVariant=Forward  IdealPFdbkVariant=Disabled  SatFdbkVariant=Disabled  DerivativeFilterVariant=Disabled  NVariant=Disabled  NCopyVariant=Disabled_SignalSpec  FilterICVariant=Disabled  IntegratorICVariant=InternalICs  ExternalResetVariant=Disabled  TRSumVariant=Passthrough  SumFdbkVariant=Disabled  SumVariant=Sum_PI
  PLL (3ph) : powerlib_meascontrol/PLL/PLL (3ph)  Fmin=55  Par_Init="[-0.57  60]"  ParK=[180, 3200, 1]  TcD=1e-4  MaxRateChangeFreq=12  FilterCutOffFreq=25  Ts=Ts_Power  AGC=on
      settings: SourceProductName=Simscape Electrical
  P_B1 : Scope  Commented=on  NumInputPorts=2
  Power (Positive-Sequence) : powerlib_meascontrol/Measurements/Power (Positive-Sequence)  Commented=on  Freq=60  Vinit=[0, 0]  Iinit=[0, 0]  Ts=Ts_Control
      settings: SourceProductName=Simscape Electrical  SourceProductBaseCode=PS
  Selector : Selector  Commented=on  InputPortWidth=3  IndexOptions=Index vector (dialog)  Indices=[1]  OutputSizes=1
  Selector1 : Selector  Commented=on  InputPortWidth=3  IndexOptions=Index vector (dialog)  Indices=[1]  OutputSizes=1
  Selector2 : Selector  InputPortWidth=3  IndexOptions=Index vector (dialog)  Indices=[1 2]  OutputSizes=1
  Selector3 : Selector  InputPortWidth=3  IndexOptions=Index vector (dialog)  Indices=[1 2]  OutputSizes=1
  Series RLC Branch : powerlib/Elements/Series RLC Branch  Commented=on  LConnTagsString=__new0  RConnTagsString=__new0  BranchType=L  Resistance=1  Inductance=1.5e-6  SetiL0=off  InitialCurrent=0  Capacitance=1e-6  Setx0=off  InitialVoltage=0  Measurements=None
      settings: SourceProductName=Simscape Electrical
  Series RLC Branch1 : powerlib/Elements/Series RLC Branch  Commented=on  LConnTagsString=__new0  RConnTagsString=__new0  BranchType=R  Resistance=3.2  Inductance=1e-3  SetiL0=off  InitialCurrent=0  Capacitance=1200e-6  Setx0=off  InitialVoltage=400  Measurements=None
      settings: SourceProductName=Simscape Electrical
  Series RLC Branch4 : powerlib/Elements/Series RLC Branch  LConnTagsString=__new0  RConnTagsString=__new0  BranchType=RC  Resistance=1e-7  Inductance=1e-3  SetiL0=off  InitialCurrent=0  Capacitance=3600e-6  Setx0=off  InitialVoltage=400  Measurements=None
      settings: SourceProductName=Simscape Electrical
  Subsystem : Subsystem  Commented=on
  Sum : Sum  Inputs=|-+
  Sum3 : Sum  Commented=on  Inputs=|-+
  Terminator : Terminator
  Terminator1 : Terminator
  Three-Phase Breaker : powerlib/Elements/Three-Phase Breaker  InitialState=open  SwitchA=on  SwitchB=on  SwitchC=on  SwitchTimes="[1/6  5/6]"  External=on  BreakerResistance=0.01e-3  SnubberResistance=30  SnubberCapacitance=20e-6  Measurements=None
      settings: SourceProductName=Simscape Electrical
  VSC (Average Model) : powerlib/Power Electronics/Universal Bridge  Arms=3  SnubberResistance=1e5  SnubberCapacitance=inf  Device=Average-model based VSC  Ron=1e-3  Lon=0  ForwardVoltages="[  0  0  ]"  ForwardVoltage=0  GTOparameters=[ 10e-6 , 20e-6 ]  IGBTparameters=[ 1e-6 , 2e-6 ]  Measurements=None  Measurements_2=None  converterType=Rectifier
      settings: SourceProductName=Simscape Electrical
  VSC (Average Model)1 : powerlib/Power Electronics/Universal Bridge  Commented=on  Arms=2  SnubberResistance=1e5  SnubberCapacitance=inf  Device=Average-model based VSC  Ron=1e-3  Lon=0  ForwardVoltages="[  0  0  ]"  ForwardVoltage=0  GTOparameters=[ 10e-6 , 20e-6 ]  IGBTparameters=[ 1e-6 , 2e-6 ]  Measurements=None  Measurements_2=None  converterType=Rectifier
      settings: SourceProductName=Simscape Electrical
  VSC (Average Model)2 : powerlib/Power Electronics/Universal Bridge  Commented=on  Arms=2  SnubberResistance=1e5  SnubberCapacitance=inf  Device=Average-model based VSC  Ron=1e-3  Lon=0  ForwardVoltages="[  0  0  ]"  ForwardVoltage=0  GTOparameters=[ 10e-6 , 20e-6 ]  IGBTparameters=[ 1e-6 , 2e-6 ]  Measurements=None  Measurements_2=None  converterType=Rectifier
      settings: SourceProductName=Simscape Electrical
  V_I grid : Scope  Commented=on  NumInputPorts=2
  Vdc_bus1 : Scope
  Voltage Measurement1 : powerlib/Measurements/Voltage Measurement  PhasorSimulation=off  OutputType=Complex  PSBequivalent=0
      settings: SourceProductName=Simscape Electrical
  W2kW : Gain  Commented=on  Gain=1/1000
  W2kW1 : Gain  Commented=on  Gain=1/1000
  abc to dq0 : powerlib_meascontrol/Transformations/abc to dq0  Alignment=90 degrees behind phase A axis
      settings: SourceProductName=Simscape Electrical
  abc to dq1 : powerlib_meascontrol/Transformations/abc to dq0  Alignment=90 degrees behind phase A axis
      settings: SourceProductName=Simscape Electrical
  dq0 to abc : powerlib_meascontrol/Transformations/dq0 to abc  Alignment=90 degrees behind phase A axis
      settings: SourceProductName=Simscape Electrical
  a : PMIOPort  Side=Right
  b : PMIOPort  Port=2  Side=Right
  c : PMIOPort  Port=3  Side=Right
  Out1 : Outport
  Qcap : Outport  Port=2
  Pcap : Outport  Port=3
  wires:
  PLL (3ph)/2 -> abc to dq1/2, abc to dq0/2, dq0 to abc/2
  Subsystem/1(Uref_DAB1) -> VSC (Average Model)2/1
  PI/1 -> Mux3/1
  Selector/1 -> V_I grid/1  "Va (V)"
  dq0 to abc/1 -> Gain/1
  Vdc_bus_ref/1 -> Sum3/2
  PLL (3ph)/1 -> Terminator/1
  From2/1 -> Selector1/1, Power (Positive-Sequence)/2
  abc to dq1/1 -> Selector2/1
  Mux3/1 -> dq0 to abc/1
  Gain/1 -> VSC (Average Model)/1
  W2kW1/1 -> P_B1/2  "Q (kVA)"
  Selector2/1 -> Sum/1
  Sum/1 -> PI/1
  [Vabc_B2_EV3] -> abc to dq0/1, PLL (3ph)/1
  Subsystem/2(Uref_DAB2) -> VSC (Average Model)1/1
  Sum3/1 -> PI3/1
  W2kW/1 -> P_B1/1  "P (kW)"
  Constant2/1 -> Mux3/2
  PI3/1 -> Subsystem/1(phase shift (-90,90))
  Selector3/1 -> Demux/1
  From3/1 -> Selector/1, Power (Positive-Sequence)/1
  Selector1/1 -> V_I grid/2
  From4/1 -> Sum3/1
  abc to dq0/1 -> Selector3/1
  Power (Positive-Sequence)/1 -> W2kW/1
  Voltage Measurement1/1 -> Vdc_bus1/1, [Vdc_EV3]
  Mux2/1 -> Sum/2
  [Iabc_B1_EV3] -> abc to dq1/1
  Power (Positive-Sequence)/2 -> W2kW1/1
  Battery/1 -> Out1/1  "Battery"
  on-off breaker/1 -> Three-Phase Breaker/1
  Demux/2 -> Terminator1/1
  Demux/1 -> [Vd_EV3]
  MATLAB Function/1(id) -> Mux2/1
  MATLAB Function/2(iq) -> Mux2/2
  [Vd_EV3] -> MATLAB Function/3(vd)
  P/1 -> MATLAB Function/1(P)  "P"
  Q/1 -> MATLAB Function/2(Q)  "Q"
  Constant1/1 -> Pcap/1
  Constant/1 -> Qcap/1
  connections:
  Battery/LConn1 -- VSC (Average Model)1/RConn1
  Three-Phase Breaker/LConn1 -- B1/RConn1
  Three-Phase Breaker/RConn2 -- B2/LConn2
  VSC (Average Model)/RConn2 -- Series RLC Branch1/RConn1 -- Voltage Measurement1/LConn2 -- Series RLC Branch4/RConn1 -- DC Voltage Source/LConn1 -- VSC (Average Model)2/RConn2
  L/RConn3 -- B1/LConn3
  L/LConn1 -- VSC (Average Model)/LConn1
  L/RConn1 -- B1/LConn1
  L/LConn2 -- VSC (Average Model)/LConn2
  Series RLC Branch1/LConn1 -- VSC (Average Model)/RConn1 -- DC Voltage Source/RConn1 -- VSC (Average Model)2/RConn1 -- Series RLC Branch4/LConn1 -- Voltage Measurement1/LConn1
  Series RLC Branch/RConn1 -- Linear Transformer/LConn1
  Linear Transformer/LConn2 -- VSC (Average Model)1/LConn2
  Three-Phase Breaker/LConn2 -- B1/RConn2
  VSC (Average Model)1/RConn2 -- Battery/LConn2
  Three-Phase Breaker/RConn3 -- B2/LConn3
  Three-Phase Breaker/RConn1 -- B2/LConn1
  Linear Transformer/RConn1 -- VSC (Average Model)2/LConn1
  Linear Transformer/RConn2 -- VSC (Average Model)2/LConn2
  c/RConn1 -- B2/RConn3
  Series RLC Branch/LConn1 -- VSC (Average Model)1/LConn1
  L/RConn2 -- B1/LConn2
  L/LConn3 -- VSC (Average Model)/LConn3
  Three-Phase Breaker/LConn3 -- B1/RConn3
  b/RConn1 -- B2/RConn2
  a/RConn1 -- B2/RConn1
